simulink model "CtrPlatform_RobustControl"  (Simulink 7.9)
settings: Solver=ode3  StartTime=0.0  StopTime=4  FixedStep=Ts  RelTol=1e-3
InitFcn:
  | eval('CtrPlatformCfg')
StopFcn:
  | eval('CtrPlotTrj')
values from neighbouring files (symbols this model uses):
  A = [a1 a2 a3 a4 a5 a6]/180*pi    [Config.m]    (also in CtrPlatformCfg.m)
  a2 = 0    [Config.m]    (also in CtrPlatformCfg.m)
  a3 = 0    [Config.m]    (also in CtrPlatformCfg.m)
  a4 = 0    [Config.m]    (also in CtrPlatformCfg.m)
  a5 = 90    [Config.m]    (also in CtrPlatformCfg.m)
  a6 = 0    [Config.m]    (also in CtrPlatformCfg.m)
  Cen = Cen(:)'    [Config.m]    (also in CtrPlatformCfg.m; DynEulerTest.m = Cen'; EfDynCAD.m = [cen1,cen2,cen3,cen4,cen5,cen6]')
  CurPulseFreq = 0.25*2*pi    (= 1.57079632679)    [Config.m]    (also in CtrPlatformCfg.m)
  Deg2Rad = pi/180    (= 0.0174532925199)    [Config.m]    (also in CtrPlatformCfg.m)
  DisturbSelect = 2    [Config.m]    (also in CtrPlatformCfg.m)
  DynTrjMode = 3    [Config.m]    (also in CtrPlatformCfg.m = 1)
  FbDisturbSelect = 2    [Config.m]    (also in CtrPlatformCfg.m)
  freq = tvel/radius    (= 1)    [Config.m]    (also in CtrPlatformCfg.m)
  FrictionSelect = 2    [CtrPlatformCfg.m]
  Gravity = 9.8    [Config.m]    (also in CtrPlatformCfg.m)
  Ie1 = in1(:)'    [Config.m]    (also in CtrPlatformCfg.m; DynEulerTest.m = in1(:); EfDynCAD.m = in1(:))
  Ie2 = in2(:)'    [Config.m]    (also in CtrPlatformCfg.m; DynEulerTest.m = in2(:); EfDynCAD.m = in2(:))
  Ie3 = in3(:)'    [Config.m]    (also in CtrPlatformCfg.m; DynEulerTest.m = in3(:); EfDynCAD.m = in3(:))
  Ie4 = in4(:)'    [Config.m]    (also in CtrPlatformCfg.m; DynEulerTest.m = in4(:); EfDynCAD.m = in4(:))
  Ie5 = in5(:)'    [Config.m]    (also in CtrPlatformCfg.m; DynEulerTest.m = in5(:); EfDynCAD.m = in5(:))
  Ie6 = in6(:)'    [Config.m]    (also in CtrPlatformCfg.m; DynEulerTest.m = in6(:); EfDynCAD.m = in6(:))
  in1 = [5.2954 -0.2565 -0.6366;-0.2565 4.7000 0.2830;-0.6366 0.2829 5.8635]    [Config.m]    (also in CtrPlatformCfg.m; DynEulerTest.m; EfDynCAD.m = [0.54  -0.01 0.23)
  in2 = [5.8840 0.0072 0.0135;0.0072 6.0178 -0.1907;0.0135 -0.1907 0.3374]    [Config.m]    (also in CtrPlatformCfg.m; DynEulerTest.m; EfDynCAD.m = (R_x*R_z)*in2*(R_x*R_z)')
  in3 = [1.8201 -0.2274 -0.3112;-0.2274 2.2537 -0.1441;-0.3112 -0.1441 1.9485]    [Config.m]    (also in CtrPlatformCfg.m; DynEulerTest.m; EfDynCAD.m = (R_x*R_z)*in3*(R_x*R_z)')
  in4 = [0.0607 -0.0922 0;-0.0922 1.4493 0;0 0 1.4620]    [Config.m]    (also in CtrPlatformCfg.m; DynEulerTest.m = [0.0607 -0.0922 0;-0.0922 1.4493 0;0 0,1.4620]; EfDynCAD.m = (R_y*Rz)*in4*(R_y*Rz)')
  in5 = [0.0191 0.0032 0;0.0032 0.0228 0;0 0 0.0291]    [Config.m]    (also in CtrPlatformCfg.m; DynEulerTest.m; EfDynCAD.m = (R_x*R_y)*in5*(R_x*R_y)')
  in6 = [0.0012 0 0;0 0.0007 0;0 0 0.0007]    [Config.m]    (also in CtrPlatformCfg.m; DynEulerTest.m; EfDynCAD.m = (R_y*Rz)*in6*(R_y*Rz)')
  init_Endx = gd_init(1,4)    [Config.m]    (also in CtrPlatformCfg.m)
  init_Endy = gd_init(2,4)    [Config.m]    (also in CtrPlatformCfg.m)
  init_Endz = gd_init(3,4)    [Config.m]    (also in CtrPlatformCfg.m)
  init_Rot = gd_init(1:3,1:3)    [Config.m]    (also in CtrPlatformCfg.m)
  InitialPos1 = A(1)*Rad2Line(1)    [CtrPlatformCfg.m]
  InitialPos2 = A(2)*Rad2Line(2)    [CtrPlatformCfg.m]
  InitialPos3 = A(3)*Rad2Line(3)    [CtrPlatformCfg.m]
  InitialPos4 = A(4)*Rad2Line(4)    [CtrPlatformCfg.m]
  InitialPos5 = A(5)*Rad2Line(5)    [CtrPlatformCfg.m]
  InitialPos6 = A(6)*Rad2Line(6)    [CtrPlatformCfg.m]
  JntOffset1 = A(1)    [Config.m]    (also in CtrPlatformCfg.m)
  JntOffset2 = A(2)    [Config.m]    (also in CtrPlatformCfg.m)
  JntOffset3 = A(3)    [Config.m]    (also in CtrPlatformCfg.m)
  JntOffset4 = A(4)    [Config.m]    (also in CtrPlatformCfg.m)
  JntOffset5 = A(5)    [Config.m]    (also in CtrPlatformCfg.m)
  JntOffset6 = A(6)    [Config.m]    (also in CtrPlatformCfg.m)
  L = [l1 l2 l3 l4 l5 l6 l7 l8 l9]    [Config.m]    (also in CtrPlatformCfg.m)
  LinePTs2RadpS = 2*pi/(EncRes*Ts)./Gear    [Config.m]    (also in CtrPlatformCfg.m)
  LinePTs2Rpm = 60/(EncRes*Ts)    (= 7.32421875)    [Config.m]    (also in CtrPlatformCfg.m)
  Ma = [ma1 ma2 ma3 ma4 ma5 ma6]    [Config.m]    (also in CtrPlatformCfg.m; DynEulerTest.m = [ma1; ma2; ma3; ma4; ma5; ma6]; EfDynCAD.m = [ma1 ma2 ma3 ma4 ma5 ma6]')
  ma1 = 170.31    [Config.m]    (also in CtrPlatformCfg.m; DynEulerTest.m; EfDynCAD.m = 77.75)
  ma2 = 63.74    [Config.m]    (also in CtrPlatformCfg.m; DynEulerTest.m; EfDynCAD.m = 32.31)
  ma3 = 98.98    [Config.m]    (also in CtrPlatformCfg.m; DynEulerTest.m; EfDynCAD.m = 18.61)
  ma4 = 24.46    [Config.m]    (also in CtrPlatformCfg.m; DynEulerTest.m; EfDynCAD.m = 15.65)
  ma5 = 5.24    [Config.m]    (also in CtrPlatformCfg.m; DynEulerTest.m; EfDynCAD.m = 3.32)
  ma6 = 0.6    [Config.m]    (also in CtrPlatformCfg.m; DynEulerTest.m; EfDynCAD.m)
  PosPulseEnable = 1    [Config.m]    (also in CtrPlatformCfg.m)
  PosSourceSelect_Ro = 2    [CtrPlatformCfg.m]
  PosVelPulseGain = 500    [Config.m]    (also in CtrPlatformCfg.m)
  Rad2Line = Gear*EncRes/(2*pi)    [Config.m]    (also in CtrPlatformCfg.m)
  Rpm2LinePTs = EncRes*Ts/60    (= 0.136533333333)    [Config.m]    (also in CtrPlatformCfg.m)
  TrajSwitch = 1    [Config.m]    (also in CtrPlatformCfg.m)
  Trq2Cur = Trq2Cur./Cur2Trq    [Config.m]    (also in CtrPlatformCfg.m)
  Ts = 1/FrHz    (= 0.00025)    [Config.m]    (also in CtrPlatformCfg.m)
  Ts_Dyn = Ts    (= 0.00025)    [Config.m]    (also in CtrPlatformCfg.m)
  tvel = 120    [Config.m]    (also in CtrPlatformCfg.m)
  VelLpAxisNum = 1    [Config.m]    (also in CtrPlatformCfg.m)
  VelPulseEnable = 0    [Config.m]    (also in CtrPlatformCfg.m)
  VelPulseGain = 500    [Config.m]    (also in CtrPlatformCfg.m)
  Volt2Trq = Volt2Trq./Trq2Cur    [Config.m]    (also in CtrPlatformCfg.m)
undefined symbols (not defined in the file or in its folder): a1, DiscIntNeverNeededParam
libraries: simulink x55, mblibv1 x35, powerlib_extras x8, commnoisgen2 x2
(part 3 of 4)

== system CtrPlatform_RobustControl/Friction Torque/Friction Torque/Ff3 ==
  dq : Inport
  Constant : Constant  Value=0  SampleTime=Ts
  Discrete-Time Integrator : DiscreteIntegrator  SampleTime=Ts  ICPrevOutput=DiscIntNeverNeededParam  ICPrevScaledInput=DiscIntNeverNeededParam
  Fp : Subsystem  mask{Ts=Ts, B1=-0.0052, B2=0.0018, B3=0.0024, B4=-0.0092}
      mask prompts: Ts "Sampling Time"
  FpSelect : Constant  Value=FpSelect  SampleTime=Ts
  Fv : Subsystem  mask{Ts=Ts, fc=50, fs=68.6, lamda=1, theta=0.0014, dqs=10}
      mask prompts: Ts "Sampling Time"
  Multiport Switch : MultiPortSwitch  Inputs=2  zeroidx=off  SampleTime=Ts
  Sum : Sum  Inputs=+|+  SampleTime=Ts
  Ff : Outport
  wires:
  Fv/1(Fv) -> Sum/2
  Multiport Switch/1 -> Sum/1
  Fp/1(Fp) -> Multiport Switch/2
  Constant/1 -> Multiport Switch/3
  FpSelect/1 -> Multiport Switch/1
  Sum/1 -> Ff/1
  Discrete-Time Integrator/1 -> Fp/1(q)
  dq/1 -> Fv/1(dq), Discrete-Time Integrator/1

== system CtrPlatform_RobustControl/Friction Torque/Friction Torque/Ff4 ==
  dq : Inport
  Constant : Constant  Value=0  SampleTime=Ts
  Discrete-Time Integrator : DiscreteIntegrator  SampleTime=Ts  ICPrevOutput=DiscIntNeverNeededParam  ICPrevScaledInput=DiscIntNeverNeededParam
  Fp : Subsystem  mask{Ts=Ts, B1=-0.0052, B2=0.0018, B3=0.0024, B4=-0.0092}
      mask prompts: Ts "Sampling Time"
  FpSelect : Constant  Value=FpSelect  SampleTime=Ts
  Fv : Subsystem  mask{Ts=Ts, fc=0.0194, fs=0.0293, lamda=2, theta=0.000013, dqs=55.219}
      mask prompts: Ts "Sampling Time"
  Multiport Switch : MultiPortSwitch  Inputs=2  zeroidx=off  SampleTime=Ts
  Sum : Sum  Inputs=+|+  SampleTime=Ts
  Ff : Outport
  wires:
  Fv/1(Fv) -> Sum/2
  Multiport Switch/1 -> Sum/1
  Fp/1(Fp) -> Multiport Switch/2
  Constant/1 -> Multiport Switch/3
  FpSelect/1 -> Multiport Switch/1
  Sum/1 -> Ff/1
  Discrete-Time Integrator/1 -> Fp/1(q)
  dq/1 -> Fv/1(dq), Discrete-Time Integrator/1

== system CtrPlatform_RobustControl/Friction Torque/Friction Torque/Ff5 ==
  dq : Inport
  Constant : Constant  Value=0  SampleTime=Ts
  Discrete-Time Integrator : DiscreteIntegrator  SampleTime=Ts  ICPrevOutput=DiscIntNeverNeededParam  ICPrevScaledInput=DiscIntNeverNeededParam
  Fp : Subsystem  mask{Ts=Ts, B1=-0.0052, B2=0.0018, B3=0.0024, B4=-0.0092}
      mask prompts: Ts "Sampling Time"
  FpSelect : Constant  Value=FpSelect  SampleTime=Ts
  Fv : Subsystem  mask{Ts=Ts, fc=0.0194, fs=0.0293, lamda=2, theta=0.000013, dqs=55.219}
      mask prompts: Ts "Sampling Time"
  Multiport Switch : MultiPortSwitch  Inputs=2  zeroidx=off  SampleTime=Ts
  Sum : Sum  Inputs=+|+  SampleTime=Ts
  Ff : Outport
  wires:
  Fv/1(Fv) -> Sum/2
  Multiport Switch/1 -> Sum/1
  Fp/1(Fp) -> Multiport Switch/2
  Constant/1 -> Multiport Switch/3
  FpSelect/1 -> Multiport Switch/1
  Sum/1 -> Ff/1
  Discrete-Time Integrator/1 -> Fp/1(q)
  dq/1 -> Fv/1(dq), Discrete-Time Integrator/1

== system CtrPlatform_RobustControl/Friction Torque/Friction Torque/Ff6 ==
  dq : Inport
  Constant : Constant  Value=0  SampleTime=Ts
  Discrete-Time Integrator : DiscreteIntegrator  SampleTime=Ts  ICPrevOutput=DiscIntNeverNeededParam  ICPrevScaledInput=DiscIntNeverNeededParam
  Fp : Subsystem  mask{Ts=Ts, B1=-0.0052, B2=0.0018, B3=0.0024, B4=-0.0092}
      mask prompts: Ts "Sampling Time"
  FpSelect : Constant  Value=FpSelect  SampleTime=Ts
  Fv : Subsystem  mask{Ts=Ts, fc=0.0194, fs=0.0293, lamda=2, theta=0.000013, dqs=55.219}
      mask prompts: Ts "Sampling Time"
  Multiport Switch : MultiPortSwitch  Inputs=2  zeroidx=off  SampleTime=Ts
  Sum : Sum  Inputs=+|+  SampleTime=Ts
  Ff : Outport
  wires:
  Fv/1(Fv) -> Sum/2
  Multiport Switch/1 -> Sum/1
  Fp/1(Fp) -> Multiport Switch/2
  Constant/1 -> Multiport Switch/3
  FpSelect/1 -> Multiport Switch/1
  Sum/1 -> Ff/1
  Discrete-Time Integrator/1 -> Fp/1(q)
  dq/1 -> Fv/1(dq), Discrete-Time Integrator/1

== system CtrPlatform_RobustControl/Trajectory Generator/Circle in Descartes Space/EndVelocity ==
  Constant : Constant  Value=-1  SampleTime=Ts_Dyn
  End_Vx : Sin  Amplitude=-tvel  Frequency=freq  SampleTime=Ts_Dyn
  End_Vy : Sin  Frequency=freq  Phase=pi/2  SampleTime=Ts_Dyn
  End_Vz : Constant  Value=0  SampleTime=Ts_Dyn
  Gain : Gain  Gain=tvel
  Integer Delay : Delay  DelayLength=1/Ts_Dyn
  Integer Delay1 : Delay  DelayLength=1/Ts_Dyn
  Ramp : simulink/Sources/Ramp  slope=1  start=0  X0=0
  Ramp1 : simulink/Sources/Ramp  slope=-1  start=1  X0=0
  Rate Transition1 : RateTransition  OutPortSampleTime=Ts_Dyn
  Rate Transition2 : RateTransition  OutPortSampleTime=Ts_Dyn
  Sum : Sum  Inputs=|++  SampleTime=Ts_Dyn
  Sum1 : Sum  Inputs=++|  SampleTime=Ts_Dyn
  Sum2 : Sum  Inputs=++|
  EndVx : Outport
  EndVy : Outport  Port=2
  EndVz : Outport  Port=3
  wires:
  End_Vy/1 -> Sum2/1
  Ramp/1 -> Rate Transition2/1
  Ramp1/1 -> Rate Transition1/1
  Integer Delay1/1 -> Sum1/1
  Sum2/1 -> Integer Delay1/1
  Constant/1 -> Sum2/2
  Sum/1 -> Sum1/2
  Sum1/1 -> Gain/1
  End_Vx/1 -> Integer Delay/1
  End_Vz/1 -> EndVx/1
  Gain/1 -> EndVy/1
  Integer Delay/1 -> EndVz/1
  Rate Transition1/1 -> Sum/2
  Rate Transition2/1 -> Sum/1

== system CtrPlatform_RobustControl/Trajectory Generator/Circle in Descartes Space/Re-group  ==
  JJVVAA : Inport
  Demux2 : Demux  Outputs=18
  Mux{,1..2,4..6} (6 alike) : Mux  Inputs=3
  Mux3 : Mux  Inputs=6
  JVAJVA : Outport
  wires:
  JJVVAA/1 -> Demux2/1
  Mux3/1 -> JVAJVA/1
  Mux/1 -> Mux3/1
  Mux1/1 -> Mux3/2
  Mux2/1 -> Mux3/3
  Mux4/1 -> Mux3/4
  Mux5/1 -> Mux3/5
  Mux6/1 -> Mux3/6
  Demux2/1 -> Mux/1
  Demux2/2 -> Mux1/1
  Demux2/3 -> Mux2/1
  Demux2/4 -> Mux4/1
  Demux2/5 -> Mux5/1
  Demux2/6 -> Mux6/1
  Demux2/7 -> Mux/2
  Demux2/8 -> Mux1/2
  Demux2/9 -> Mux2/2
  Demux2/10 -> Mux4/2
  Demux2/11 -> Mux5/2
  Demux2/12 -> Mux6/2
  Demux2/13 -> Mux/3
  Demux2/14 -> Mux1/3
  Demux2/15 -> Mux2/3
  Demux2/16 -> Mux4/3
  Demux2/17 -> Mux5/3
  Demux2/18 -> Mux6/3

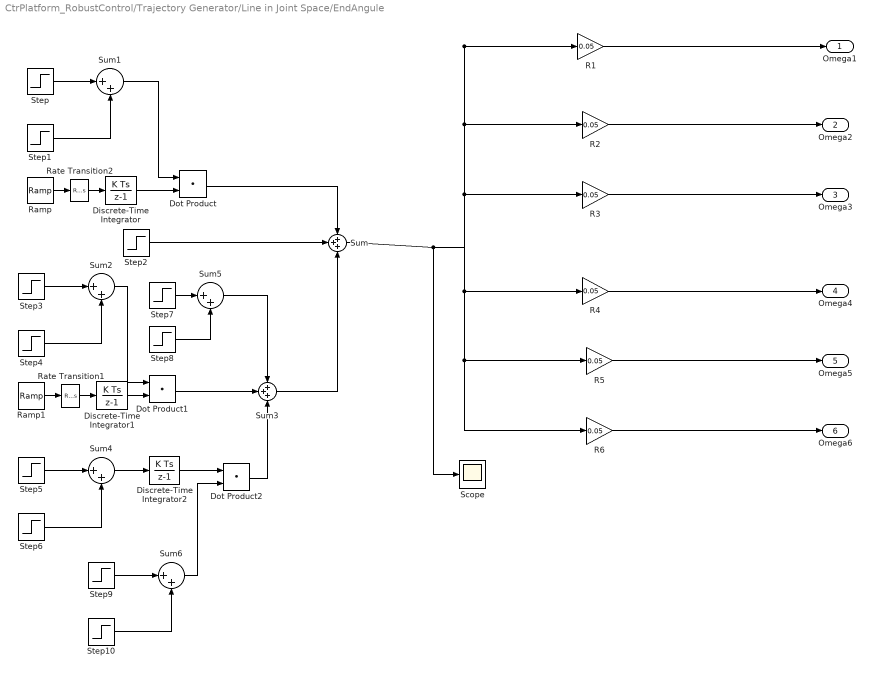
== system CtrPlatform_RobustControl/Trajectory Generator/Line in Joint Space/EndAngule ==
  Discrete-Time Integrator : DiscreteIntegrator  SampleTime=Ts_Dyn  ICPrevOutput=DiscIntNeverNeededParam  ICPrevScaledInput=DiscIntNeverNeededParam
  Discrete-Time Integrator1 : DiscreteIntegrator  SampleTime=Ts_Dyn  ICPrevOutput=DiscIntNeverNeededParam  ICPrevScaledInput=DiscIntNeverNeededParam
  Discrete-Time Integrator2 : DiscreteIntegrator  SampleTime=Ts_Dyn  ICPrevOutput=DiscIntNeverNeededParam  ICPrevScaledInput=DiscIntNeverNeededParam
  Dot Product : DotProduct  InputSameDT=on  OutDataTypeStr=Inherit: Inherit via internal rule
  Dot Product1 : DotProduct  InputSameDT=on  OutDataTypeStr=Inherit: Inherit via internal rule
  Dot Product2 : DotProduct  InputSameDT=on  OutDataTypeStr=Inherit: Inherit via internal rule
  R{1..6} (6 alike) : Gain  Gain=0.05
  Ramp : simulink/Sources/Ramp  slope=1  start=0  X0=0
  Ramp1 : simulink/Sources/Ramp  slope=-1  start=0  X0=0
  Rate Transition1 : RateTransition  OutPortSampleTime=Ts_Dyn
  Rate Transition2 : RateTransition  OutPortSampleTime=Ts_Dyn
  Scope : Scope
      settings: SaveName=ScopeData21
  Step : Step  After=-1  SampleTime=Ts_Dyn
  Step1 : Step  Time=0  SampleTime=Ts_Dyn
  Step10 : Step  SampleTime=Ts_Dyn
  Step2 : Step  Time=2  SampleTime=Ts_Dyn
  Step3 : Step  Time=2  After=-1  SampleTime=Ts_Dyn
  Step4 : Step  SampleTime=Ts_Dyn
  Step5 : Step  Time=2  After=-2  SampleTime=Ts_Dyn
  Step6 : Step  After=2  SampleTime=Ts_Dyn
  Step7 : Step  Time=2  After=-1  SampleTime=Ts_Dyn
  Step8 : Step  SampleTime=Ts_Dyn
  Step9 : Step  Time=2  After=-1  SampleTime=Ts_Dyn
  Sum : Sum  Inputs=+++
  Sum{1..2,4..6} (5 alike) : Sum  Inputs=|++
  Sum3 : Sum  Inputs=+++
  Omega1 : Outport
  Omega2 : Outport  Port=2
  Omega3 : Outport  Port=3
  Omega4 : Outport  Port=4
  Omega5 : Outport  Port=5
  Omega6 : Outport  Port=6
  wires:
  R4/1 -> Omega4/1
  R6/1 -> Omega6/1
  R5/1 -> Omega5/1
  R3/1 -> Omega3/1
  R2/1 -> Omega2/1
  Ramp/1 -> Rate Transition2/1
  R1/1 -> Omega1/1
  Sum/1 -> R1/1, R2/1, R3/1, R4/1, R5/1, R6/1, Scope/1
  Discrete-Time Integrator/1 -> Dot Product/2
  Step/1 -> Sum1/1
  Sum1/1 -> Dot Product/1
  Step1/1 -> Sum1/2
  Dot Product/1 -> Sum/1
  Step2/1 -> Sum/2
  Ramp1/1 -> Rate Transition1/1
  Discrete-Time Integrator1/1 -> Dot Product1/2
  Step3/1 -> Sum2/1
  Sum2/1 -> Dot Product1/1
  Step4/1 -> Sum2/2
  Sum3/1 -> Sum/3
  Step5/1 -> Sum4/1
  Step6/1 -> Sum4/2
  Sum4/1 -> Discrete-Time Integrator2/1
  Dot Product1/1 -> Sum3/2
  Step7/1 -> Sum5/1
  Step8/1 -> Sum5/2
  Sum5/1 -> Sum3/1
  Step9/1 -> Sum6/1
  Step10/1 -> Sum6/2
  Discrete-Time Integrator2/1 -> Dot Product2/1
  Sum6/1 -> Dot Product2/2
  Dot Product2/1 -> Sum3/3
  Rate Transition1/1 -> Discrete-Time Integrator1/1
  Rate Transition2/1 -> Discrete-Time Integrator/1

== system CtrPlatform_RobustControl/Trajectory Generator/Line in Joint Space/Re-group  ==
  JJVVAA : Inport
  Demux2 : Demux  Outputs=18
  Mux{,1..2,4..6} (6 alike) : Mux  Inputs=3
  Mux3 : Mux  Inputs=6
  JVAJVA : Outport
  wires:
  JJVVAA/1 -> Demux2/1
  Mux3/1 -> JVAJVA/1
  Mux/1 -> Mux3/1
  Mux1/1 -> Mux3/2
  Mux2/1 -> Mux3/3
  Mux4/1 -> Mux3/4
  Mux5/1 -> Mux3/5
  Mux6/1 -> Mux3/6
  Demux2/1 -> Mux/1
  Demux2/2 -> Mux1/1
  Demux2/3 -> Mux2/1
  Demux2/4 -> Mux4/1
  Demux2/5 -> Mux5/1
  Demux2/6 -> Mux6/1
  Demux2/7 -> Mux/2
  Demux2/8 -> Mux1/2
  Demux2/9 -> Mux2/2
  Demux2/10 -> Mux4/2
  Demux2/11 -> Mux5/2
  Demux2/12 -> Mux6/2
  Demux2/13 -> Mux/3
  Demux2/14 -> Mux1/3
  Demux2/15 -> Mux2/3
  Demux2/16 -> Mux4/3
  Demux2/17 -> Mux5/3
  Demux2/18 -> Mux6/3

== system CtrPlatform_RobustControl/Trajectory Generator/Still/EndVelocity ==
  Constant : Constant  Value=0  SampleTime=Ts_Dyn
  Constant1 : Constant  Value=0  SampleTime=Ts_Dyn
  Constant2 : Constant  Value=0  SampleTime=Ts_Dyn
  EndVx : Outport
  EndVy : Outport  Port=2
  EndVz : Outport  Port=3
  wires:
  Constant/1 -> EndVx/1
  Constant1/1 -> EndVy/1
  Constant2/1 -> EndVz/1

== system CtrPlatform_RobustControl/Trajectory Generator/Still/Re-group  ==
  JJVVAA : Inport
  Demux2 : Demux  Outputs=18
  Mux{,1..2,4..6} (6 alike) : Mux  Inputs=3
  Mux3 : Mux  Inputs=6
  JVAJVA : Outport
  wires:
  Demux2/18 -> Mux6/3
  Demux2/17 -> Mux5/3
  Demux2/16 -> Mux4/3
  Demux2/15 -> Mux2/3
  Demux2/14 -> Mux1/3
  Demux2/13 -> Mux/3
  Demux2/12 -> Mux6/2
  Demux2/11 -> Mux5/2
  Demux2/10 -> Mux4/2
  Demux2/9 -> Mux2/2
  Demux2/8 -> Mux1/2
  Demux2/7 -> Mux/2
  Demux2/6 -> Mux6/1
  Demux2/5 -> Mux5/1
  Demux2/4 -> Mux4/1
  Demux2/3 -> Mux2/1
  Demux2/2 -> Mux1/1
  Demux2/1 -> Mux/1
  Mux6/1 -> Mux3/6
  Mux5/1 -> Mux3/5
  Mux4/1 -> Mux3/4
  Mux2/1 -> Mux3/3
  Mux1/1 -> Mux3/2
  Mux/1 -> Mux3/1
  Mux3/1 -> JVAJVA/1
  JJVVAA/1 -> Demux2/1

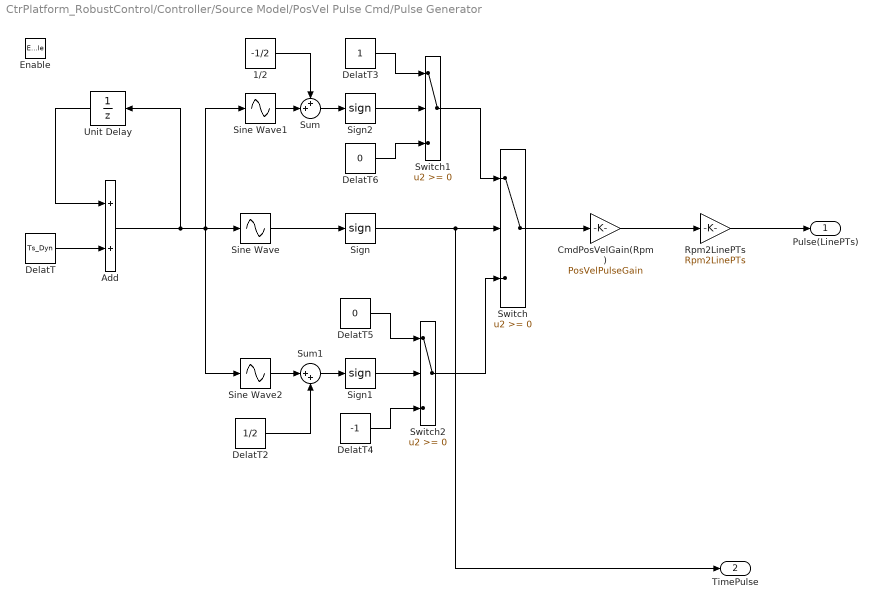
== system CtrPlatform_RobustControl/Controller/Source Model/PosVel Pulse Cmd/Pulse Generator ==
  Enable : EnablePort
  1/2 : Constant  Value=-1/2  SampleTime=Ts_Dyn
  Add : Sum
  CmdPosVelGain(Rpm) : Gain  Gain=PosVelPulseGain
  DelatT : Constant  Value=Ts_Dyn  SampleTime=Ts_Dyn
  DelatT2 : Constant  Value=1/2  SampleTime=Ts_Dyn
  DelatT3 : Constant  SampleTime=Ts_Dyn
  DelatT4 : Constant  Value=-1  SampleTime=Ts_Dyn
  DelatT5 : Constant  Value=0  SampleTime=Ts_Dyn
  DelatT6 : Constant  Value=0  SampleTime=Ts_Dyn
  Rpm2LinePTs : Gain  Gain=Rpm2LinePTs
  Sign : Signum
  Sign1 : Signum
  Sign2 : Signum
  Sine Wave : Sin  TimeSource=Use external signal  Frequency=CurPulseFreq  SampleTime=0
  Sine Wave1 : Sin  TimeSource=Use external signal  Frequency=0.25*2*pi  SampleTime=0
  Sine Wave2 : Sin  TimeSource=Use external signal  Frequency=0.25*2*pi  SampleTime=0
  Sum : Sum  Inputs=++|
  Sum1 : Sum  Inputs=|++
  Switch : Switch
  Switch1 : Switch
  Switch2 : Switch
  Unit Delay : UnitDelay  SampleTime=Ts_Dyn
  Pulse(LinePTs) : Outport
  TimePulse : Outport  Port=2
  wires:
  Rpm2LinePTs/1 -> Pulse(LinePTs)/1
  CmdPosVelGain(Rpm)/1 -> Rpm2LinePTs/1
  Sine Wave/1 -> Sign/1
  DelatT/1 -> Add/2
  Unit Delay/1 -> Add/1
  Add/1 -> Unit Delay/1, Sine Wave/1, Sine Wave1/1, Sine Wave2/1
  Sign/1 -> Switch/2, TimePulse/1
  Switch/1 -> CmdPosVelGain(Rpm)/1
  Switch1/1 -> Switch/1
  Switch2/1 -> Switch/3
  Sine Wave1/1 -> Sum/2
  1/2/1 -> Sum/1
  Sine Wave2/1 -> Sum1/1
  DelatT2/1 -> Sum1/2
  Sum1/1 -> Sign1/1
  Sign1/1 -> Switch2/2
  Sum/1 -> Sign2/1
  Sign2/1 -> Switch1/2
  DelatT3/1 -> Switch1/1
  DelatT4/1 -> Switch2/3
  DelatT5/1 -> Switch2/1
  DelatT6/1 -> Switch1/3

== system CtrPlatform_RobustControl/Controller/Source Model/PosVel Pulse Cmd/Triggered Subsystem ==
  Trigger : TriggerPort
  One : Constant  OutDataTypeStr=boolean  SampleTime=-1
  Out1 : Outport
  wires:
  One/1 -> Out1/1

== system CtrPlatform_RobustControl/Controller/Source Model/PosVel Pulse Cmd/Zero Refrence ==
  Enable : EnablePort
  Bias : Constant  Value=0  SampleTime=Ts_Dyn
  Pulse : Outport
  wires:
  Bias/1 -> Pulse/1

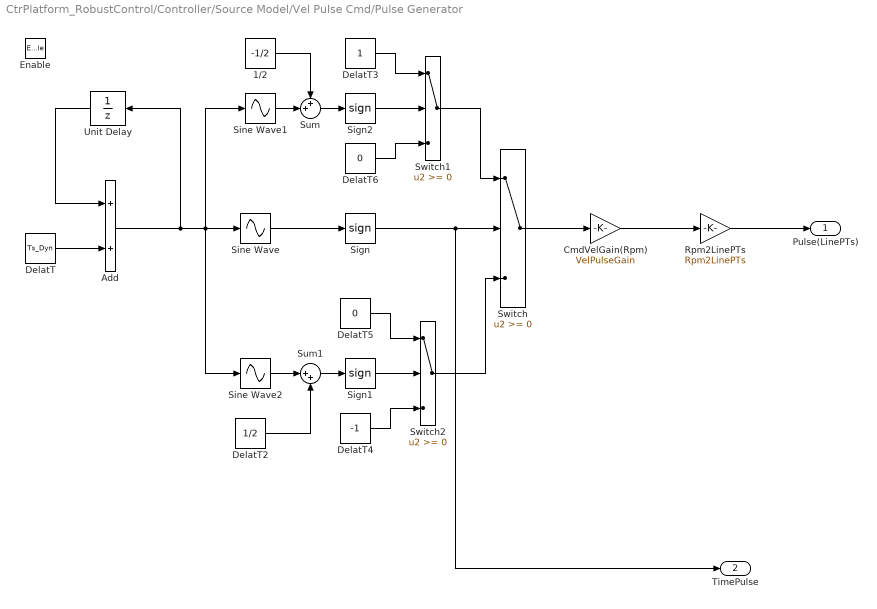
== system CtrPlatform_RobustControl/Controller/Source Model/Vel Pulse Cmd/Pulse Generator ==
  Enable : EnablePort
  1/2 : Constant  Value=-1/2  SampleTime=Ts_Dyn
  Add : Sum
  CmdVelGain(Rpm) : Gain  Gain=VelPulseGain
  DelatT : Constant  Value=Ts_Dyn  SampleTime=Ts_Dyn
  DelatT2 : Constant  Value=1/2  SampleTime=Ts_Dyn
  DelatT3 : Constant  SampleTime=Ts_Dyn
  DelatT4 : Constant  Value=-1  SampleTime=Ts_Dyn
  DelatT5 : Constant  Value=0  SampleTime=Ts_Dyn
  DelatT6 : Constant  Value=0  SampleTime=Ts_Dyn
  Rpm2LinePTs : Gain  Gain=Rpm2LinePTs
  Sign : Signum
  Sign1 : Signum
  Sign2 : Signum
  Sine Wave : Sin  TimeSource=Use external signal  Frequency=CurPulseFreq  SampleTime=0
  Sine Wave1 : Sin  TimeSource=Use external signal  Frequency=0.25*2*pi  SampleTime=0
  Sine Wave2 : Sin  TimeSource=Use external signal  Frequency=0.25*2*pi  SampleTime=0
  Sum : Sum  Inputs=++|
  Sum1 : Sum  Inputs=|++
  Switch : Switch
  Switch1 : Switch
  Switch2 : Switch
  Unit Delay : UnitDelay  SampleTime=Ts_Dyn
  Pulse(LinePTs) : Outport
  TimePulse : Outport  Port=2
  wires:
  DelatT6/1 -> Switch1/3
  DelatT5/1 -> Switch2/1
  DelatT4/1 -> Switch2/3
  DelatT3/1 -> Switch1/1
  Sign2/1 -> Switch1/2
  Sum/1 -> Sign2/1
  Sign1/1 -> Switch2/2
  Sum1/1 -> Sign1/1
  DelatT2/1 -> Sum1/2
  Sine Wave2/1 -> Sum1/1
  1/2/1 -> Sum/1
  Sine Wave1/1 -> Sum/2
  Switch2/1 -> Switch/3
  Switch1/1 -> Switch/1
  Switch/1 -> CmdVelGain(Rpm)/1
  Sign/1 -> TimePulse/1, Switch/2
  Add/1 -> Sine Wave2/1, Sine Wave1/1, Sine Wave/1, Unit Delay/1
  Unit Delay/1 -> Add/1
  DelatT/1 -> Add/2
  Sine Wave/1 -> Sign/1
  CmdVelGain(Rpm)/1 -> Rpm2LinePTs/1
  Rpm2LinePTs/1 -> Pulse(LinePTs)/1

== system CtrPlatform_RobustControl/Controller/Source Model/Vel Pulse Cmd/Triggered Subsystem ==
  Trigger : TriggerPort
  One : Constant  OutDataTypeStr=boolean  SampleTime=-1
  Out1 : Outport
  wires:
  One/1 -> Out1/1

== system CtrPlatform_RobustControl/Controller/Source Model/Vel Pulse Cmd/Zero Refrence ==
  Enable : EnablePort
  Bias : Constant  Value=0  SampleTime=Ts_Dyn
  Pulse : Outport
  wires:
  Bias/1 -> Pulse/1

== system CtrPlatform_RobustControl/Dynamics/TrjSource/Position Loop Tunning/Axis1 ==
  Discrete Derivative : simulink/Discrete/Discrete Derivative  gainval=1.0  ICPrevScaledInput=0.0  InputProcessing=Inherited  OutMin=[]  OutMax=[]  OutDataType=sfix(16)  OutScaling=2^-10  DoSatur=off
  Discrete-Time Integrator : DiscreteIntegrator  SampleTime=-1  ICPrevOutput=DiscIntNeverNeededParam  ICPrevScaledInput=DiscIntNeverNeededParam
  JntOffset1 : Constant  Value=JntOffset1
  JntOffset2 : Constant  Value=JntOffset2
  JntOffset3 : Constant  Value=JntOffset3
  JntOffset4 : Constant  Value=JntOffset4
  JntOffset5 : Constant  Value=JntOffset5
  JntOffset6 : Constant  Value=JntOffset6
  LinePTs2RadpS : Gain  Gain=LinePTs2RadpS(1)
  Mux : Mux  Inputs=6
  Mux1 : Mux  Inputs=6
  Mux2 : Mux  Inputs=6
  Sum : Sum  Inputs=++|
  Zero : Constant  Value=0
  JntPos(Rad) : Outport
  JntVel(Rad/s) : Outport  Port=2
  JntAcc(Rad/s2) : Outport  Port=3
  wires:
  LinePTs2RadpS/1 -> Mux1/1, Discrete-Time Integrator/1, Discrete Derivative/1
  Mux2/1 -> JntAcc(Rad/s2)/1
  Mux1/1 -> JntVel(Rad/s)/1
  Mux/1 -> JntPos(Rad)/1
  Zero/1 -> Mux1/2, Mux1/3, Mux1/4, Mux1/5, Mux1/6, Mux2/2, Mux2/3, Mux2/4, Mux2/5, Mux2/6
  JntOffset6/1 -> Mux/6
  JntOffset5/1 -> Mux/5
  JntOffset4/1 -> Mux/4
  JntOffset3/1 -> Mux/3
  JntOffset2/1 -> Mux/2
  JntOffset1/1 -> Sum/1
  Sum/1 -> Mux/1
  Discrete-Time Integrator/1 -> Sum/2
  Discrete Derivative/1 -> Mux2/1
  [PosVel_Pulse_Dyn] -> LinePTs2RadpS/1

== system CtrPlatform_RobustControl/Dynamics/TrjSource/Position Loop Tunning/Axis2 ==
  Discrete Derivative : simulink/Discrete/Discrete Derivative  gainval=1.0  ICPrevScaledInput=0.0  InputProcessing=Inherited  OutMin=[]  OutMax=[]  OutDataType=sfix(16)  OutScaling=2^-10  DoSatur=off
  Discrete-Time Integrator : DiscreteIntegrator  SampleTime=-1  ICPrevOutput=DiscIntNeverNeededParam  ICPrevScaledInput=DiscIntNeverNeededParam
  JntOffset1 : Constant  Value=JntOffset1
  JntOffset2 : Constant  Value=JntOffset2
  JntOffset3 : Constant  Value=JntOffset3
  JntOffset4 : Constant  Value=JntOffset4
  JntOffset5 : Constant  Value=JntOffset5
  JntOffset6 : Constant  Value=JntOffset6
  LinePTs2RadpS : Gain  Gain=LinePTs2RadpS(2)
  Mux : Mux  Inputs=6
  Mux1 : Mux  Inputs=6
  Mux2 : Mux  Inputs=6
  Sum : Sum  Inputs=++|
  Zero : Constant  Value=0
  JntPos(Rad) : Outport
  JntVel(Rad/s) : Outport  Port=2
  JntAcc(Rad/s2) : Outport  Port=3
  wires:
  LinePTs2RadpS/1 -> Mux1/2, Discrete Derivative/1, Discrete-Time Integrator/1
  Discrete Derivative/1 -> Mux2/2
  JntOffset1/1 -> Mux/1
  Sum/1 -> Mux/2
  [PosVel_Pulse_Dyn] -> LinePTs2RadpS/1
  Discrete-Time Integrator/1 -> Sum/2
  JntOffset2/1 -> Sum/1
  JntOffset3/1 -> Mux/3
  JntOffset4/1 -> Mux/4
  JntOffset5/1 -> Mux/5
  JntOffset6/1 -> Mux/6
  Zero/1 -> Mux2/6, Mux2/5, Mux2/4, Mux2/1, Mux1/6, Mux1/5, Mux1/1, Mux1/3, Mux1/4, Mux2/3
  Mux/1 -> JntPos(Rad)/1
  Mux1/1 -> JntVel(Rad/s)/1
  Mux2/1 -> JntAcc(Rad/s2)/1

== system CtrPlatform_RobustControl/Dynamics/TrjSource/Position Loop Tunning/Axis3 ==
  Discrete Derivative : simulink/Discrete/Discrete Derivative  gainval=1.0  ICPrevScaledInput=0.0  InputProcessing=Inherited  OutMin=[]  OutMax=[]  OutDataType=sfix(16)  OutScaling=2^-10  DoSatur=off
  Discrete-Time Integrator : DiscreteIntegrator  SampleTime=-1  ICPrevOutput=DiscIntNeverNeededParam  ICPrevScaledInput=DiscIntNeverNeededParam
  JntOffset1 : Constant  Value=JntOffset1
  JntOffset2 : Constant  Value=JntOffset2
  JntOffset3 : Constant  Value=JntOffset3
  JntOffset4 : Constant  Value=JntOffset4
  JntOffset5 : Constant  Value=JntOffset5
  JntOffset6 : Constant  Value=JntOffset6
  LinePTs2RadpS : Gain  Gain=LinePTs2RadpS(3)
  Mux : Mux  Inputs=6
  Mux1 : Mux  Inputs=6
  Mux2 : Mux  Inputs=6
  Sum : Sum  Inputs=++|
  Zero : Constant  Value=0
  JntPos(Rad) : Outport
  JntVel(Rad/s) : Outport  Port=2
  JntAcc(Rad/s2) : Outport  Port=3
  wires:
  LinePTs2RadpS/1 -> Mux1/3, Discrete Derivative/1, Discrete-Time Integrator/1
  Discrete Derivative/1 -> Mux2/3
  JntOffset1/1 -> Mux/1
  Sum/1 -> Mux/3
  Mux2/1 -> JntAcc(Rad/s2)/1
  Mux1/1 -> JntVel(Rad/s)/1
  Mux/1 -> JntPos(Rad)/1
  Zero/1 -> Mux2/1, Mux1/1, Mux1/2, Mux1/4, Mux1/5, Mux1/6, Mux2/2, Mux2/4, Mux2/5, Mux2/6
  JntOffset6/1 -> Mux/6
  JntOffset5/1 -> Mux/5
  JntOffset4/1 -> Mux/4
  JntOffset2/1 -> Mux/2
  JntOffset3/1 -> Sum/1
  Discrete-Time Integrator/1 -> Sum/2
  [PosVel_Pulse_Dyn] -> LinePTs2RadpS/1

== system CtrPlatform_RobustControl/Dynamics/TrjSource/Position Loop Tunning/Axis4 ==
  AbsEnc4 : Constant  Value=JntOffset4
  Discrete Derivative : simulink/Discrete/Discrete Derivative  gainval=1.0  ICPrevScaledInput=0.0  InputProcessing=Inherited  OutMin=[]  OutMax=[]  OutDataType=sfix(16)  OutScaling=2^-10  DoSatur=off
  Discrete-Time Integrator : DiscreteIntegrator  SampleTime=-1  ICPrevOutput=DiscIntNeverNeededParam  ICPrevScaledInput=DiscIntNeverNeededParam
  JntOffset1 : Constant  Value=JntOffset1
  JntOffset2 : Constant  Value=JntOffset2
  JntOffset3 : Constant  Value=JntOffset3
  JntOffset5 : Constant  Value=JntOffset5
  JntOffset6 : Constant  Value=JntOffset6
  LinePTs2RadpS : Gain  Gain=LinePTs2RadpS(4)
  Mux : Mux  Inputs=6
  Mux1 : Mux  Inputs=6
  Mux2 : Mux  Inputs=6
  Sum : Sum  Inputs=++|
  Zero : Constant  Value=0
  JntPos(Rad) : Outport
  JntVel(Rad/s) : Outport  Port=2
  JntAcc(Rad/s2) : Outport  Port=3
  wires:
  LinePTs2RadpS/1 -> Mux1/4, Discrete Derivative/1, Discrete-Time Integrator/1
  Sum/1 -> Mux/4
  JntOffset1/1 -> Mux/1
  [PosVel_Pulse_Dyn] -> LinePTs2RadpS/1
  Discrete Derivative/1 -> Mux2/1
  Discrete-Time Integrator/1 -> Sum/2
  AbsEnc4/1 -> Sum/1
  JntOffset2/1 -> Mux/2
  JntOffset3/1 -> Mux/3
  JntOffset5/1 -> Mux/5
  JntOffset6/1 -> Mux/6
  Zero/1 -> Mux2/6, Mux2/5, Mux2/4, Mux2/3, Mux2/2, Mux1/6, Mux1/1, Mux1/2, Mux1/3, Mux1/5
  Mux/1 -> JntPos(Rad)/1
  Mux1/1 -> JntVel(Rad/s)/1
  Mux2/1 -> JntAcc(Rad/s2)/1

== system CtrPlatform_RobustControl/Dynamics/TrjSource/Position Loop Tunning/Axis5 ==
  Discrete Derivative : simulink/Discrete/Discrete Derivative  gainval=1.0  ICPrevScaledInput=0.0  InputProcessing=Inherited  OutMin=[]  OutMax=[]  OutDataType=sfix(16)  OutScaling=2^-10  DoSatur=off
  Discrete-Time Integratr : DiscreteIntegrator  SampleTime=-1  ICPrevOutput=DiscIntNeverNeededParam  ICPrevScaledInput=DiscIntNeverNeededParam
  JntOffset1 : Constant  Value=JntOffset1
  JntOffset2 : Constant  Value=JntOffset2
  JntOffset3 : Constant  Value=JntOffset3
  JntOffset4 : Constant  Value=JntOffset4
  JntOffset5 : Constant  Value=JntOffset5
  JntOffset6 : Constant  Value=JntOffset6
  LinePTs2RadpS : Gain  Gain=LinePTs2RadpS(5)
  Mux : Mux  Inputs=6
  Mux1 : Mux  Inputs=6
  Mux2 : Mux  Inputs=6
  Sum : Sum  Inputs=++|
  Zero : Constant  Value=0
  JntPos(Rad) : Outport
  JntVel(Rad/s) : Outport  Port=2
  JntAcc(Rad/s2) : Outport  Port=3
  wires:
  LinePTs2RadpS/1 -> Mux1/5, Discrete Derivative/1, Discrete-Time Integratr/1
  Discrete Derivative/1 -> Mux2/5
  Sum/1 -> Mux/5
  JntOffset1/1 -> Mux/1
  Mux2/1 -> JntAcc(Rad/s2)/1
  Mux1/1 -> JntVel(Rad/s)/1
  Mux/1 -> JntPos(Rad)/1
  Zero/1 -> Mux2/1, Mux1/1, Mux1/2, Mux1/3, Mux1/4, Mux1/6, Mux2/2, Mux2/3, Mux2/4, Mux2/6
  JntOffset6/1 -> Mux/6
  JntOffset4/1 -> Mux/4
  JntOffset3/1 -> Mux/3
  JntOffset2/1 -> Mux/2
  JntOffset5/1 -> Sum/1
  Discrete-Time Integratr/1 -> Sum/2
  [PosVel_Pulse_Dyn] -> LinePTs2RadpS/1

== system CtrPlatform_RobustControl/Dynamics/TrjSource/Position Loop Tunning/Axis6 ==
  Discrete Derivative : simulink/Discrete/Discrete Derivative  gainval=1.0  ICPrevScaledInput=0.0  InputProcessing=Inherited  OutMin=[]  OutMax=[]  OutDataType=sfix(16)  OutScaling=2^-10  DoSatur=off
  Discrete-Time Integrator : DiscreteIntegrator  SampleTime=-1  ICPrevOutput=DiscIntNeverNeededParam  ICPrevScaledInput=DiscIntNeverNeededParam
  JntOffset1 : Constant  Value=JntOffset1
  JntOffset2 : Constant  Value=JntOffset2
  JntOffset3 : Constant  Value=JntOffset3
  JntOffset4 : Constant  Value=JntOffset4
  JntOffset5 : Constant  Value=JntOffset5
  JntOffset6 : Constant  Value=JntOffset6
  LinePTs2RadpS : Gain  Gain=LinePTs2RadpS(6)
  Mux : Mux  Inputs=6
  Mux1 : Mux  Inputs=6
  Mux2 : Mux  Inputs=6
  Sum : Sum  Inputs=++|
  Zero : Constant  Value=0
  JntPos(Rad) : Outport
  JntVel(Rad/s) : Outport  Port=2
  JntAcc(Rad/s2) : Outport  Port=3
  wires:
  LinePTs2RadpS/1 -> Mux1/6, Discrete Derivative/1, Discrete-Time Integrator/1
  Discrete Derivative/1 -> Mux2/6
  JntOffset1/1 -> Mux/1
  Sum/1 -> Mux/6
  [PosVel_Pulse_Dyn] -> LinePTs2RadpS/1
  Discrete-Time Integrator/1 -> Sum/2
  JntOffset6/1 -> Sum/1
  JntOffset2/1 -> Mux/2
  JntOffset3/1 -> Mux/3
  JntOffset4/1 -> Mux/4
  JntOffset5/1 -> Mux/5
  Zero/1 -> Mux2/5, Mux2/4, Mux2/3, Mux2/2, Mux1/5, Mux1/4, Mux1/1, Mux1/2, Mux1/3, Mux2/1
  Mux/1 -> JntPos(Rad)/1
  Mux1/1 -> JntVel(Rad/s)/1
  Mux2/1 -> JntAcc(Rad/s2)/1

== system CtrPlatform_RobustControl/Dynamics/TrjSource/Velocity Loop Tunning/Axis1 ==
  Discrete Derivative : simulink/Discrete/Discrete Derivative  gainval=1.0  ICPrevScaledInput=0.0  InputProcessing=Inherited  OutMin=[]  OutMax=[]  OutDataType=sfix(16)  OutScaling=2^-10  DoSatur=off
  Discrete-Time Integrator : DiscreteIntegrator  SampleTime=-1  ICPrevOutput=DiscIntNeverNeededParam  ICPrevScaledInput=DiscIntNeverNeededParam
  JntOffset1 : Constant  Value=JntOffset1  SampleTime=Ts_Dyn
  JntOffset2 : Constant  Value=JntOffset2  SampleTime=Ts_Dyn
  JntOffset3 : Constant  Value=JntOffset3  SampleTime=Ts_Dyn
  JntOffset4 : Constant  Value=JntOffset4  SampleTime=Ts_Dyn
  JntOffset5 : Constant  Value=JntOffset5  SampleTime=Ts_Dyn
  JntOffset6 : Constant  Value=JntOffset6  SampleTime=Ts_Dyn
  LinePTs2RadpS : Gain  Gain=LinePTs2RadpS(1)
  Mux : Mux  Inputs=6
  Mux1 : Mux  Inputs=6
  Mux2 : Mux  Inputs=6
  Sum : Sum  Inputs=++|
  Zero : Constant  Value=0  SampleTime=Ts_Dyn
  JntPos(Rad) : Outport
  JntVel(Rad/s) : Outport  Port=2
  JntAcc(Rad/s2) : Outport  Port=3
  wires:
  [Vel_Pulse_Dyn] -> LinePTs2RadpS/1
  Discrete Derivative/1 -> Mux2/1
  Sum/1 -> Mux/1
  JntOffset1/1 -> Sum/1
  JntOffset2/1 -> Mux/2
  JntOffset3/1 -> Mux/3
  JntOffset4/1 -> Mux/4
  JntOffset5/1 -> Mux/5
  JntOffset6/1 -> Mux/6
  Zero/1 -> Mux2/6, Mux2/5, Mux2/4, Mux2/3, Mux2/2, Mux1/6, Mux1/5, Mux1/4, Mux1/3, Mux1/2
  Mux/1 -> JntPos(Rad)/1
  Mux1/1 -> JntVel(Rad/s)/1
  Mux2/1 -> JntAcc(Rad/s2)/1
  LinePTs2RadpS/1 -> Discrete Derivative/1, Mux1/1, Discrete-Time Integrator/1
  Discrete-Time Integrator/1 -> Sum/2

== system CtrPlatform_RobustControl/Dynamics/TrjSource/Velocity Loop Tunning/Axis2 ==
  Discrete Derivative : simulink/Discrete/Discrete Derivative  gainval=1.0  ICPrevScaledInput=0.0  InputProcessing=Inherited  OutMin=[]  OutMax=[]  OutDataType=sfix(16)  OutScaling=2^-10  DoSatur=off
  Discrete-Time Integrator : DiscreteIntegrator  SampleTime=-1  ICPrevOutput=DiscIntNeverNeededParam  ICPrevScaledInput=DiscIntNeverNeededParam
  JntOffset1 : Constant  Value=JntOffset1  SampleTime=Ts_Dyn
  JntOffset2 : Constant  Value=JntOffset2  SampleTime=Ts_Dyn
  JntOffset3 : Constant  Value=JntOffset3  SampleTime=Ts_Dyn
  JntOffset4 : Constant  Value=JntOffset4  SampleTime=Ts_Dyn
  JntOffset5 : Constant  Value=JntOffset5  SampleTime=Ts_Dyn
  JntOffset6 : Constant  Value=JntOffset6  SampleTime=Ts_Dyn
  LinePTs2RadpS : Gain  Gain=LinePTs2RadpS(2)
  Mux : Mux  Inputs=6
  Mux1 : Mux  Inputs=6
  Mux2 : Mux  Inputs=6
  Sum : Sum  Inputs=++|
  Zero : Constant  Value=0  SampleTime=Ts_Dyn
  JntPos(Rad) : Outport
  JntVel(Rad/s) : Outport  Port=2
  JntAcc(Rad/s2) : Outport  Port=3
  wires:
  Mux2/1 -> JntAcc(Rad/s2)/1
  Mux1/1 -> JntVel(Rad/s)/1
  Mux/1 -> JntPos(Rad)/1
  Zero/1 -> Mux2/3, Mux1/4, Mux1/3, Mux1/1, Mux1/5, Mux1/6, Mux2/1, Mux2/4, Mux2/5, Mux2/6
  JntOffset6/1 -> Mux/6
  JntOffset5/1 -> Mux/5
  JntOffset4/1 -> Mux/4
  JntOffset3/1 -> Mux/3
  JntOffset2/1 -> Sum/1
  Discrete-Time Integrator/1 -> Sum/2
  [Vel_Pulse_Dyn] -> LinePTs2RadpS/1
  Sum/1 -> Mux/2
  JntOffset1/1 -> Mux/1
  Discrete Derivative/1 -> Mux2/2
  LinePTs2RadpS/1 -> Discrete-Time Integrator/1, Discrete Derivative/1, Mux1/2

== system CtrPlatform_RobustControl/Dynamics/TrjSource/Velocity Loop Tunning/Axis3 ==
  Discrete Derivative : simulink/Discrete/Discrete Derivative  gainval=1.0  ICPrevScaledInput=0.0  InputProcessing=Inherited  OutMin=[]  OutMax=[]  OutDataType=sfix(16)  OutScaling=2^-10  DoSatur=off
  Discrete-Time Integrator : DiscreteIntegrator  SampleTime=-1  ICPrevOutput=DiscIntNeverNeededParam  ICPrevScaledInput=DiscIntNeverNeededParam
  JntOffset1 : Constant  Value=JntOffset1  SampleTime=Ts_Dyn
  JntOffset2 : Constant  Value=JntOffset2  SampleTime=Ts_Dyn
  JntOffset3 : Constant  Value=JntOffset3  SampleTime=Ts_Dyn
  JntOffset4 : Constant  Value=JntOffset4  SampleTime=Ts_Dyn
  JntOffset5 : Constant  Value=JntOffset5  SampleTime=Ts_Dyn
  JntOffset6 : Constant  Value=JntOffset6  SampleTime=Ts_Dyn
  LinePTs2RadpS : Gain  Gain=LinePTs2RadpS(3)
  Mux : Mux  Inputs=6
  Mux1 : Mux  Inputs=6
  Mux2 : Mux  Inputs=6
  Sum : Sum  Inputs=++|
  Zero : Constant  Value=0  SampleTime=Ts_Dyn
  JntPos(Rad) : Outport
  JntVel(Rad/s) : Outport  Port=2
  JntAcc(Rad/s2) : Outport  Port=3
  wires:
  [Vel_Pulse_Dyn] -> LinePTs2RadpS/1
  Discrete-Time Integrator/1 -> Sum/2
  JntOffset3/1 -> Sum/1
  JntOffset2/1 -> Mux/2
  JntOffset4/1 -> Mux/4
  JntOffset5/1 -> Mux/5
  JntOffset6/1 -> Mux/6
  Zero/1 -> Mux2/6, Mux2/5, Mux2/4, Mux2/2, Mux1/6, Mux1/5, Mux1/4, Mux1/2, Mux1/1, Mux2/1
  Mux/1 -> JntPos(Rad)/1
  Mux1/1 -> JntVel(Rad/s)/1
  Mux2/1 -> JntAcc(Rad/s2)/1
  Sum/1 -> Mux/3
  JntOffset1/1 -> Mux/1
  Discrete Derivative/1 -> Mux2/3
  LinePTs2RadpS/1 -> Discrete-Time Integrator/1, Discrete Derivative/1, Mux1/3

== system CtrPlatform_RobustControl/Dynamics/TrjSource/Velocity Loop Tunning/Axis4 ==
  AbsEnc4 : Constant  Value=JntOffset4  SampleTime=Ts_Dyn
  Discrete Derivative : simulink/Discrete/Discrete Derivative  gainval=1.0  ICPrevScaledInput=0.0  InputProcessing=Inherited  OutMin=[]  OutMax=[]  OutDataType=sfix(16)  OutScaling=2^-10  DoSatur=off
  Discrete-Time Integrator : DiscreteIntegrator  SampleTime=-1  ICPrevOutput=DiscIntNeverNeededParam  ICPrevScaledInput=DiscIntNeverNeededParam
  JntOffset1 : Constant  Value=JntOffset1  SampleTime=Ts_Dyn
  JntOffset2 : Constant  Value=JntOffset2  SampleTime=Ts_Dyn
  JntOffset3 : Constant  Value=JntOffset3  SampleTime=Ts_Dyn
  JntOffset5 : Constant  Value=JntOffset5  SampleTime=Ts_Dyn
  JntOffset6 : Constant  Value=JntOffset6  SampleTime=Ts_Dyn
  LinePTs2RadpS : Gain  Gain=LinePTs2RadpS(4)
  Mux : Mux  Inputs=6
  Mux1 : Mux  Inputs=6
  Mux2 : Mux  Inputs=6
  Sum : Sum  Inputs=++|
  Zero : Constant  Value=0  SampleTime=Ts_Dyn
  JntPos(Rad) : Outport
  JntVel(Rad/s) : Outport  Port=2
  JntAcc(Rad/s2) : Outport  Port=3
  wires:
  Mux2/1 -> JntAcc(Rad/s2)/1
  Mux1/1 -> JntVel(Rad/s)/1
  Mux/1 -> JntPos(Rad)/1
  Zero/1 -> Mux1/5, Mux1/3, Mux1/2, Mux1/1, Mux1/6, Mux2/2, Mux2/3, Mux2/4, Mux2/5, Mux2/6
  JntOffset6/1 -> Mux/6
  JntOffset5/1 -> Mux/5
  JntOffset3/1 -> Mux/3
  JntOffset2/1 -> Mux/2
  AbsEnc4/1 -> Sum/1
  Discrete-Time Integrator/1 -> Sum/2
  Discrete Derivative/1 -> Mux2/1
  [Vel_Pulse_Dyn] -> LinePTs2RadpS/1
  JntOffset1/1 -> Mux/1
  Sum/1 -> Mux/4
  LinePTs2RadpS/1 -> Discrete-Time Integrator/1, Discrete Derivative/1, Mux1/4

== system CtrPlatform_RobustControl/Dynamics/TrjSource/Velocity Loop Tunning/Axis5 ==
  Discrete Derivative : simulink/Discrete/Discrete Derivative  gainval=1.0  ICPrevScaledInput=0.0  InputProcessing=Inherited  OutMin=[]  OutMax=[]  OutDataType=sfix(16)  OutScaling=2^-10  DoSatur=off
  Discrete-Time Integratr : DiscreteIntegrator  SampleTime=-1  ICPrevOutput=DiscIntNeverNeededParam  ICPrevScaledInput=DiscIntNeverNeededParam
  JntOffset1 : Constant  Value=JntOffset1  SampleTime=Ts_Dyn
  JntOffset2 : Constant  Value=JntOffset2  SampleTime=Ts_Dyn
  JntOffset3 : Constant  Value=JntOffset3  SampleTime=Ts_Dyn
  JntOffset4 : Constant  Value=JntOffset4  SampleTime=Ts_Dyn
  JntOffset5 : Constant  Value=JntOffset5  SampleTime=Ts_Dyn
  JntOffset6 : Constant  Value=JntOffset6  SampleTime=Ts_Dyn
  LinePTs2RadpS : Gain  Gain=LinePTs2RadpS(5)
  Mux : Mux  Inputs=6
  Mux1 : Mux  Inputs=6
  Mux2 : Mux  Inputs=6
  Sum : Sum  Inputs=++|
  Zero : Constant  Value=0  SampleTime=Ts_Dyn
  JntPos(Rad) : Outport
  JntVel(Rad/s) : Outport  Port=2
  JntAcc(Rad/s2) : Outport  Port=3
  wires:
  [Vel_Pulse_Dyn] -> LinePTs2RadpS/1
  Discrete-Time Integratr/1 -> Sum/2
  JntOffset5/1 -> Sum/1
  JntOffset2/1 -> Mux/2
  JntOffset3/1 -> Mux/3
  JntOffset4/1 -> Mux/4
  JntOffset6/1 -> Mux/6
  Zero/1 -> Mux2/6, Mux2/4, Mux2/3, Mux2/2, Mux1/6, Mux1/4, Mux1/3, Mux1/2, Mux1/1, Mux2/1
  Mux/1 -> JntPos(Rad)/1
  Mux1/1 -> JntVel(Rad/s)/1
  Mux2/1 -> JntAcc(Rad/s2)/1
  JntOffset1/1 -> Mux/1
  Sum/1 -> Mux/5
  Discrete Derivative/1 -> Mux2/5
  LinePTs2RadpS/1 -> Discrete-Time Integratr/1, Discrete Derivative/1, Mux1/5

== system CtrPlatform_RobustControl/Dynamics/TrjSource/Velocity Loop Tunning/Axis6 ==
  Discrete Derivative : simulink/Discrete/Discrete Derivative  gainval=1.0  ICPrevScaledInput=0.0  InputProcessing=Inherited  OutMin=[]  OutMax=[]  OutDataType=sfix(16)  OutScaling=2^-10  DoSatur=off
  Discrete-Time Integrator : DiscreteIntegrator  SampleTime=-1  ICPrevOutput=DiscIntNeverNeededParam  ICPrevScaledInput=DiscIntNeverNeededParam
  JntOffset1 : Constant  Value=JntOffset1
  JntOffset2 : Constant  Value=JntOffset2
  JntOffset3 : Constant  Value=JntOffset3
  JntOffset4 : Constant  Value=JntOffset4
  JntOffset5 : Constant  Value=JntOffset5
  JntOffset6 : Constant  Value=JntOffset6
  LinePTs2RadpS : Gain  Gain=LinePTs2RadpS(6)
  Mux : Mux  Inputs=6
  Mux1 : Mux  Inputs=6
  Mux2 : Mux  Inputs=6
  Sum : Sum  Inputs=++|
  Zero : Constant  Value=0
  JntPos(Rad) : Outport
  JntVel(Rad/s) : Outport  Port=2
  JntAcc(Rad/s2) : Outport  Port=3
  wires:
  Mux2/1 -> JntAcc(Rad/s2)/1
  Mux1/1 -> JntVel(Rad/s)/1
  Mux/1 -> JntPos(Rad)/1
  Zero/1 -> Mux2/2, Mux1/3, Mux1/2, Mux1/1, Mux1/4, Mux1/5, Mux2/1, Mux2/3, Mux2/4, Mux2/5
  JntOffset5/1 -> Mux/5
  JntOffset4/1 -> Mux/4
  JntOffset3/1 -> Mux/3
  JntOffset2/1 -> Mux/2
  JntOffset6/1 -> Sum/1
  Discrete-Time Integrator/1 -> Sum/2
  [Vel_Pulse_Dyn] -> LinePTs2RadpS/1
  Sum/1 -> Mux/6
  JntOffset1/1 -> Mux/1
  Discrete Derivative/1 -> Mux2/6
  LinePTs2RadpS/1 -> Discrete-Time Integrator/1, Discrete Derivative/1, Mux1/6

== system CtrPlatform_RobustControl/Friction Torque/Friction Torque/Ff1/Fp ==
  q : Inport
  Add : Sum  Inputs=++++  SampleTime=Ts
  B1 : Gain  Gain=B1  SampleTime=Ts
  B2 : Gain  Gain=B2  SampleTime=Ts
  B3 : Gain  Gain=B3  SampleTime=Ts
  B4 : Gain  Gain=B4  SampleTime=Ts
  Cosine : simulink/Lookup Tables/Cosine  Formula=cos(2*pi*u)  NumDataPoints=(2^5)+1  OutputWordLength=16
  Cosine1 : simulink/Lookup Tables/Cosine  Formula=cos(2*pi*u)  NumDataPoints=(2^5)+1  OutputWordLength=16
  Gain : Gain  Gain=1/(2*pi)  SampleTime=Ts
  Gain1 : Gain  Gain=1/pi  SampleTime=Ts
  Sine : simulink/Lookup Tables/Sine  Formula=sin(2*pi*u)  NumDataPoints=(2^5)+1  OutputWordLength=16
  Sine1 : simulink/Lookup Tables/Sine  Formula=sin(2*pi*u)  NumDataPoints=(2^5)+1  OutputWordLength=16
  Fp : Outport
  wires:
  Gain/1 -> Sine/1, Cosine/1
  Gain1/1 -> Sine1/1, Cosine1/1
  q/1 -> Gain/1, Gain1/1
  Cosine1/1 -> B4/1
  Sine1/1 -> B3/1
  Cosine/1 -> B2/1
  Sine/1 -> B1/1
  B2/1 -> Add/2
  B3/1 -> Add/3
  B4/1 -> Add/4
  B1/1 -> Add/1
  Add/1 -> Fp/1

== system CtrPlatform_RobustControl/Friction Torque/Friction Torque/Ff1/Fv1 ==
  dq : Inport
  Abs : Abs  SampleTime=Ts
  Add : Sum  SampleTime=Ts
  Add1 : Sum  SampleTime=Ts
  Divide : Product  Inputs=*/  SampleTime=Ts
  Gain : Constant  Value=-1  SampleTime=Ts
  Math Function : Math  Operator=pow  SampleTime=Ts  SaturateOnIntegerOverflow=on
  Math Function1 : Math  SampleTime=Ts  SaturateOnIntegerOverflow=on
  Product{,1..3} (4 alike) : Product  SampleTime=Ts  RndMeth=Zero
  Sign : Signum  SampleTime=Ts
  Subtract : Sum  Inputs=-+  SampleTime=Ts
  dqs : Constant  Value=dqs  SampleTime=Ts
  fc : Constant  Value=fc  SampleTime=Ts
  fs : Constant  Value=fs  SampleTime=Ts
  lamda : Constant  Value=lamda  SampleTime=Ts
  theta : Constant  Value=theta  SampleTime=Ts
  Fv : Outport
  wires:
  dq/1 -> Divide/1, Sign/1, Product3/2
  dqs/1 -> Divide/2
  Divide/1 -> Abs/1
  Abs/1 -> Math Function/1
  lamda/1 -> Math Function/2
  Math Function/1 -> Product/1
  Gain/1 -> Product/2
  Product/1 -> Math Function1/1
  fc/1 -> Subtract/1, Add/1
  fs/1 -> Subtract/2
  Subtract/1 -> Product1/1
  Math Function1/1 -> Product1/2
  Product1/1 -> Add/2
  Sign/1 -> Product2/1
  Add/1 -> Product2/2
  Product3/1 -> Add1/1
  Product2/1 -> Add1/2
  theta/1 -> Product3/1
  Add1/1 -> Fv/1

== system CtrPlatform_RobustControl/Friction Torque/Friction Torque/Ff2/Fp ==
  q : Inport
  Add : Sum  Inputs=++++  SampleTime=Ts
  B1 : Gain  Gain=B1  SampleTime=Ts
  B2 : Gain  Gain=B2  SampleTime=Ts
  B3 : Gain  Gain=B3  SampleTime=Ts
  B4 : Gain  Gain=B4  SampleTime=Ts
  Cosine : simulink/Lookup Tables/Cosine  Formula=cos(2*pi*u)  NumDataPoints=(2^5)+1  OutputWordLength=16
  Cosine1 : simulink/Lookup Tables/Cosine  Formula=cos(2*pi*u)  NumDataPoints=(2^5)+1  OutputWordLength=16
  Gain : Gain  Gain=1/(2*pi)  SampleTime=Ts
  Gain1 : Gain  Gain=1/pi  SampleTime=Ts
  Sine : simulink/Lookup Tables/Sine  Formula=sin(2*pi*u)  NumDataPoints=(2^5)+1  OutputWordLength=16
  Sine1 : simulink/Lookup Tables/Sine  Formula=sin(2*pi*u)  NumDataPoints=(2^5)+1  OutputWordLength=16
  Fp : Outport
  wires:
  Gain/1 -> Sine/1, Cosine/1
  Gain1/1 -> Sine1/1, Cosine1/1
  q/1 -> Gain/1, Gain1/1
  Cosine1/1 -> B4/1
  Sine1/1 -> B3/1
  Cosine/1 -> B2/1
  Sine/1 -> B1/1
  B2/1 -> Add/2
  B3/1 -> Add/3
  B4/1 -> Add/4
  B1/1 -> Add/1
  Add/1 -> Fp/1

== system CtrPlatform_RobustControl/Friction Torque/Friction Torque/Ff2/Fv ==
  dq : Inport
  Abs : Abs  SampleTime=Ts
  Add : Sum  SampleTime=Ts
  Add1 : Sum  SampleTime=Ts
  Divide : Product  Inputs=*/  SampleTime=Ts
  Gain : Constant  Value=-1  SampleTime=Ts
  Math Function : Math  Operator=pow  SampleTime=Ts  SaturateOnIntegerOverflow=on
  Math Function1 : Math  SampleTime=Ts  SaturateOnIntegerOverflow=on
  Product{,1..3} (4 alike) : Product  SampleTime=Ts  RndMeth=Zero
  Sign : Signum  SampleTime=Ts
  Subtract : Sum  Inputs=-+  SampleTime=Ts
  dqs : Constant  Value=dqs  SampleTime=Ts
  fc : Constant  Value=fc  SampleTime=Ts
  fs : Constant  Value=fs  SampleTime=Ts
  lamda : Constant  Value=lamda  SampleTime=Ts
  theta : Constant  Value=theta  SampleTime=Ts
  Fv : Outport
  wires:
  dq/1 -> Divide/1, Sign/1, Product3/2
  dqs/1 -> Divide/2
  Divide/1 -> Abs/1
  Abs/1 -> Math Function/1
  lamda/1 -> Math Function/2
  Math Function/1 -> Product/1
  Gain/1 -> Product/2
  Product/1 -> Math Function1/1
  fc/1 -> Subtract/1, Add/1
  fs/1 -> Subtract/2
  Subtract/1 -> Product1/1
  Math Function1/1 -> Product1/2
  Product1/1 -> Add/2
  Sign/1 -> Product2/1
  Add/1 -> Product2/2
  Product3/1 -> Add1/1
  Product2/1 -> Add1/2
  theta/1 -> Product3/1
  Add1/1 -> Fv/1

== system CtrPlatform_RobustControl/Friction Torque/Friction Torque/Ff3/Fp ==
  q : Inport
  Add : Sum  Inputs=++++  SampleTime=Ts
  B1 : Gain  Gain=B1  SampleTime=Ts
  B2 : Gain  Gain=B2  SampleTime=Ts
  B3 : Gain  Gain=B3  SampleTime=Ts
  B4 : Gain  Gain=B4  SampleTime=Ts
  Cosine : simulink/Lookup Tables/Cosine  Formula=cos(2*pi*u)  NumDataPoints=(2^5)+1  OutputWordLength=16
  Cosine1 : simulink/Lookup Tables/Cosine  Formula=cos(2*pi*u)  NumDataPoints=(2^5)+1  OutputWordLength=16
  Gain : Gain  Gain=1/(2*pi)  SampleTime=Ts
  Gain1 : Gain  Gain=1/pi  SampleTime=Ts
  Sine : simulink/Lookup Tables/Sine  Formula=sin(2*pi*u)  NumDataPoints=(2^5)+1  OutputWordLength=16
  Sine1 : simulink/Lookup Tables/Sine  Formula=sin(2*pi*u)  NumDataPoints=(2^5)+1  OutputWordLength=16
  Fp : Outport
  wires:
  Gain/1 -> Sine/1, Cosine/1
  Gain1/1 -> Sine1/1, Cosine1/1
  q/1 -> Gain/1, Gain1/1
  Cosine1/1 -> B4/1
  Sine1/1 -> B3/1
  Cosine/1 -> B2/1
  Sine/1 -> B1/1
  B2/1 -> Add/2
  B3/1 -> Add/3
  B4/1 -> Add/4
  B1/1 -> Add/1
  Add/1 -> Fp/1

== system CtrPlatform_RobustControl/Friction Torque/Friction Torque/Ff3/Fv ==
  dq : Inport
  Abs : Abs  SampleTime=Ts
  Add : Sum  SampleTime=Ts
  Add1 : Sum  SampleTime=Ts
  Divide : Product  Inputs=*/  SampleTime=Ts
  Gain : Constant  Value=-1  SampleTime=Ts
  Math Function : Math  Operator=pow  SampleTime=Ts  SaturateOnIntegerOverflow=on
  Math Function1 : Math  SampleTime=Ts  SaturateOnIntegerOverflow=on
  Product{,1..3} (4 alike) : Product  SampleTime=Ts  RndMeth=Zero
  Sign : Signum  SampleTime=Ts
  Subtract : Sum  Inputs=-+  SampleTime=Ts
  dqs : Constant  Value=dqs  SampleTime=Ts
  fc : Constant  Value=fc  SampleTime=Ts
  fs : Constant  Value=fs  SampleTime=Ts
  lamda : Constant  Value=lamda  SampleTime=Ts
  theta : Constant  Value=theta  SampleTime=Ts
  Fv : Outport
  wires:
  dq/1 -> Divide/1, Sign/1, Product3/2
  dqs/1 -> Divide/2
  Divide/1 -> Abs/1
  Abs/1 -> Math Function/1
  lamda/1 -> Math Function/2
  Math Function/1 -> Product/1
  Gain/1 -> Product/2
  Product/1 -> Math Function1/1
  fc/1 -> Subtract/1, Add/1
  fs/1 -> Subtract/2
  Subtract/1 -> Product1/1
  Math Function1/1 -> Product1/2
  Product1/1 -> Add/2
  Sign/1 -> Product2/1
  Add/1 -> Product2/2
  Product3/1 -> Add1/1
  Product2/1 -> Add1/2
  theta/1 -> Product3/1
  Add1/1 -> Fv/1

== system CtrPlatform_RobustControl/Friction Torque/Friction Torque/Ff4/Fp ==
  q : Inport
  Add : Sum  Inputs=++++  SampleTime=Ts
  B1 : Gain  Gain=B1  SampleTime=Ts
  B2 : Gain  Gain=B2  SampleTime=Ts
  B3 : Gain  Gain=B3  SampleTime=Ts
  B4 : Gain  Gain=B4  SampleTime=Ts
  Cosine : simulink/Lookup Tables/Cosine  Formula=cos(2*pi*u)  NumDataPoints=(2^5)+1  OutputWordLength=16
  Cosine1 : simulink/Lookup Tables/Cosine  Formula=cos(2*pi*u)  NumDataPoints=(2^5)+1  OutputWordLength=16
  Gain : Gain  Gain=1/(2*pi)  SampleTime=Ts
  Gain1 : Gain  Gain=1/pi  SampleTime=Ts
  Sine : simulink/Lookup Tables/Sine  Formula=sin(2*pi*u)  NumDataPoints=(2^5)+1  OutputWordLength=16
  Sine1 : simulink/Lookup Tables/Sine  Formula=sin(2*pi*u)  NumDataPoints=(2^5)+1  OutputWordLength=16
  Fp : Outport
  wires:
  Gain/1 -> Sine/1, Cosine/1
  Gain1/1 -> Sine1/1, Cosine1/1
  q/1 -> Gain/1, Gain1/1
  Cosine1/1 -> B4/1
  Sine1/1 -> B3/1
  Cosine/1 -> B2/1
  Sine/1 -> B1/1
  B2/1 -> Add/2
  B3/1 -> Add/3
  B4/1 -> Add/4
  B1/1 -> Add/1
  Add/1 -> Fp/1

== system CtrPlatform_RobustControl/Friction Torque/Friction Torque/Ff4/Fv ==
  dq : Inport
  Abs : Abs  SampleTime=Ts
  Add : Sum  SampleTime=Ts
  Add1 : Sum  SampleTime=Ts
  Divide : Product  Inputs=*/  SampleTime=Ts
  Gain : Constant  Value=-1  SampleTime=Ts
  Math Function : Math  Operator=pow  SampleTime=Ts  SaturateOnIntegerOverflow=on
  Math Function1 : Math  SampleTime=Ts  SaturateOnIntegerOverflow=on
  Product{,1..3} (4 alike) : Product  SampleTime=Ts  RndMeth=Zero
  Sign : Signum  SampleTime=Ts
  Subtract : Sum  Inputs=-+  SampleTime=Ts
  dqs : Constant  Value=dqs  SampleTime=Ts
  fc : Constant  Value=fc  SampleTime=Ts
  fs : Constant  Value=fs  SampleTime=Ts
  lamda : Constant  Value=lamda  SampleTime=Ts
  theta : Constant  Value=theta  SampleTime=Ts
  Fv : Outport
  wires:
  dq/1 -> Divide/1, Sign/1, Product3/2
  dqs/1 -> Divide/2
  Divide/1 -> Abs/1
  Abs/1 -> Math Function/1
  lamda/1 -> Math Function/2
  Math Function/1 -> Product/1
  Gain/1 -> Product/2
  Product/1 -> Math Function1/1
  fc/1 -> Subtract/1, Add/1
  fs/1 -> Subtract/2
  Subtract/1 -> Product1/1
  Math Function1/1 -> Product1/2
  Product1/1 -> Add/2
  Sign/1 -> Product2/1
  Add/1 -> Product2/2
  Product3/1 -> Add1/1
  Product2/1 -> Add1/2
  theta/1 -> Product3/1
  Add1/1 -> Fv/1

== system CtrPlatform_RobustControl/Friction Torque/Friction Torque/Ff5/Fp ==
  q : Inport
  Add : Sum  Inputs=++++  SampleTime=Ts
  B1 : Gain  Gain=B1  SampleTime=Ts
  B2 : Gain  Gain=B2  SampleTime=Ts
  B3 : Gain  Gain=B3  SampleTime=Ts
  B4 : Gain  Gain=B4  SampleTime=Ts
  Cosine : simulink/Lookup Tables/Cosine  Formula=cos(2*pi*u)  NumDataPoints=(2^5)+1  OutputWordLength=16
  Cosine1 : simulink/Lookup Tables/Cosine  Formula=cos(2*pi*u)  NumDataPoints=(2^5)+1  OutputWordLength=16
  Gain : Gain  Gain=1/(2*pi)  SampleTime=Ts
  Gain1 : Gain  Gain=1/pi  SampleTime=Ts
  Sine : simulink/Lookup Tables/Sine  Formula=sin(2*pi*u)  NumDataPoints=(2^5)+1  OutputWordLength=16
  Sine1 : simulink/Lookup Tables/Sine  Formula=sin(2*pi*u)  NumDataPoints=(2^5)+1  OutputWordLength=16
  Fp : Outport
  wires:
  Gain/1 -> Sine/1, Cosine/1
  Gain1/1 -> Sine1/1, Cosine1/1
  q/1 -> Gain/1, Gain1/1
  Cosine1/1 -> B4/1
  Sine1/1 -> B3/1
  Cosine/1 -> B2/1
  Sine/1 -> B1/1
  B2/1 -> Add/2
  B3/1 -> Add/3
  B4/1 -> Add/4
  B1/1 -> Add/1
  Add/1 -> Fp/1
